simulink model "yarpWriteDoubles"  (Simulink 7.3)
settings: Solver=ode45  SolverMode=SingleTasking  StartTime=0.0  StopTime=inf  RelTol=1e-3  AbsTol=1e-6
libraries: simulink x1, utility x1
settings Model: Creator=dmedonza  LastModifiedBy=yo
settings DataIOCC: SaveOutput=off  SignalLogging=off  SaveTime=off
settings OptimizationCC: BooleanDataType=off
settings DebuggingCC: SaveWithParameterizedLinksMsg=none  SignalResolutionControl=TryResolveAllWithWarning  SolverPrmCheckMsg=none  MultiTaskDSMMsg=warning  MultiTaskCondExecSysMsg=none  StrictBusMsg=None
settings HardwareCC: TargetUnknown=on
settings RTWCC: TemplateMakefile=grt_vc.tmf  IncludeERTFirstTime=on

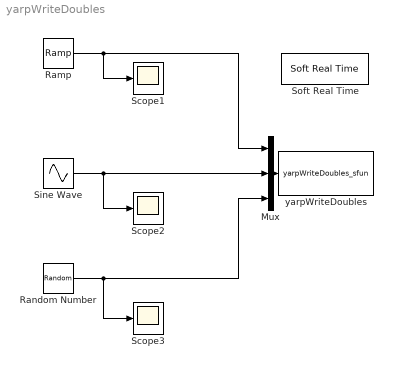
== system yarpWriteDoubles ==
  Mux : Mux  Inputs=3
  Ramp : simulink/Sources/Ramp  SystemSampleTime=-1  slope=1  start=0  X0=0
  Random Number : RandomNumber  SampleTime=0.1
  Scope1 : Scope
      settings: TimeRange=10  YMin=0  YMax=8
  Scope2 : Scope
      settings: YMin=-1  YMax=1
  Scope3 : Scope
      settings: YMin=-2.5  YMax=2.5  SaveName=ScopeData2
  Sine Wave : Sin  Amplitude=1  Bias=0  Frequency=1  Phase=0  Samples=10  SampleTime=0  Offset=0
  Soft Real Time : utility/Soft Real Time  x=1
  yarpWriteDoubles : S-Function  FunctionName=yarpWriteDoubles_sfun  Parameters=setNumDoubles  EnableBusSupport=off  mask{setNumDoubles=3}
      mask prompts: setNumDoubles "Number of Doubles"
      mask help: The yarpWriteDoubles block tries to open a YARP port called /yarpWriteDoubles, connect to a port called /read, and then stream some doubles!!!
      mask Display: image(imread('yarpPipes.png'))
  wires:
  Ramp/1 -> Mux/1, Scope1/1
  Mux/1 -> yarpWriteDoubles/1
  Sine Wave/1 -> Mux/2, Scope2/1
  Random Number/1 -> Mux/3, Scope3/1
